simulink model "gyroPendulumBall"  (R2018a)
settings: Solver=FixedStepDiscrete  StartTime=0.0  StopTime=inf  FixedStep=timeStep  RelTol=1e-3
values from neighbouring files (symbols this model uses):
  K1 = [K1(1, :) K1(2, :)]    [alphaParallel.m]    (also in setup.m = lqr(Aw1, Bw1, diag([1, 1, 3, 1, 1, 1]), diag([6, 6])))
  K2 = lqr(Aw2, Bw2, diag([15, 1, 1, 5]), diag([15]))    [setup.m]
  K3 = lqr(Aw3, Bw3, diag([1, 1, 1, 1]), diag([1]))    [setup.m]
  modelParameters = rmfield(modelParameters, 'alph2')    [alphaParallel.m]    (also in setup.m)
  trajectory = [0.204039137261 -0.389047482528 0.184950739835 -0.34807965922 0.208093560422 -0.397377880713 0.182464301801 -0.343183800683 0.212362955443 -0.406162696705 0.180157605825 -0.338633761035 ... (832 elements, 4x208)]    [trajectory.mat]
  trajectoryTimeStep = 0.005    [setup.m]
  trajectoryToWalk = [0.20348839193 -0.387921068139 0.185314050902 -0.348794213842 0.206937106898 -0.395034683488 0.18313781068 -0.34450971149 0.210555704125 -0.402555806913 0.181086396317 -0.340463307968 ... (484 elements, 4x121)]    [trajectoryToWalk.mat]
  trajectoryWalk = [0.250192072849 -0.608547594051 0.394694165643 -0.613804432575 0.251033796696 -0.60716129389 0.397031433715 -0.614641196656 0.251771384595 -0.605603254171 0.399919372114 -0.616088285913 ... (1104 elements, 4x276)]    [trajectoryWalk.mat]
undefined symbols (not defined in the file or in its folder): DiscIntNeverNeededParam
libraries: simulink x4, dspindex x3, sharedtransform x1
settings Model: EnablePacing=on  PacingRate=2  Creator=Oleg  LastModifiedBy=sorok

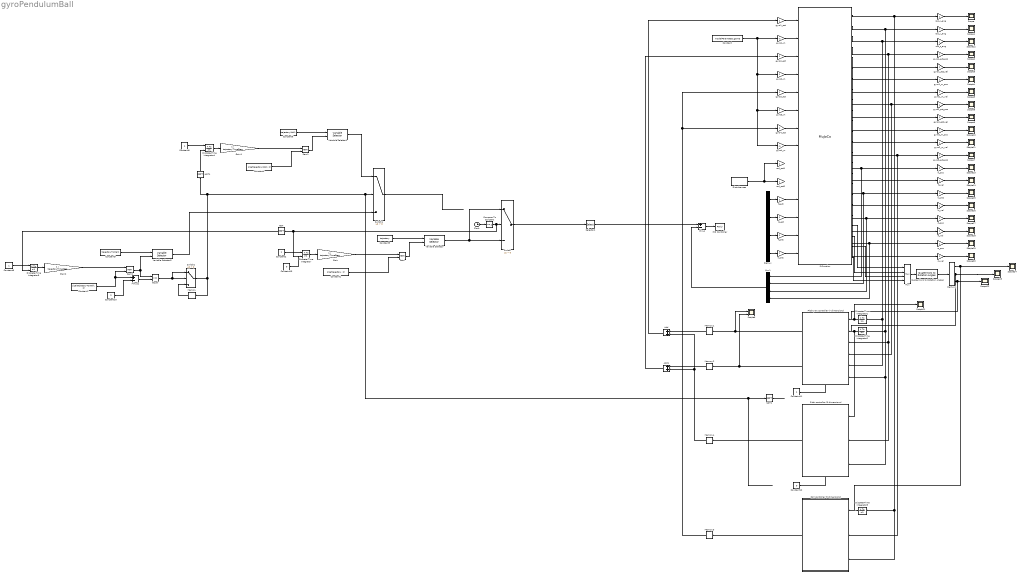
== system gyroPendulumBall ==
  Add : Sum
  Add1 : Sum
  Clock : Clock
  Compare To Constant : simulink/Logic and Bit Operations/Compare To Constant  relop=>=  const=2  OutDataTypeStr=boolean
  Constant : Constant  Value=modelParameters.gamD
  Constant1 : Constant  Value=size(trajectory, 2)
  Constant10 : Constant  Value=2
  Constant11 : Constant
  Constant12 : Constant  Value=0
  Constant13 : Constant  Value=0
  Constant2 : Constant  SampleTime=trajectoryTimeStep
  Constant3 : Constant  Value=trajectory
  Constant4 : Constant  Value=size(trajectoryWalk, 2)
  Constant5 : Constant  SampleTime=trajectoryTimeStep
  Constant6 : Constant  Value=trajectoryWalk
  Constant7 : Constant  Value=size(trajectoryToWalk, 2)
  Constant8 : Constant  SampleTime=trajectoryTimeStep
  Constant9 : Constant  Value=trajectoryToWalk
  Demux : Demux
  Demux1 : Demux  Outputs=3
  Discrete-Time Integrator : DiscreteIntegrator  ExternalReset=level  SampleTime=-1  ICPrevOutput=DiscIntNeverNeededParam  ICPrevScaledInput=DiscIntNeverNeededParam
  Discrete-Time Integrator1 : DiscreteIntegrator  SampleTime=-1  ICPrevOutput=DiscIntNeverNeededParam  ICPrevScaledInput=DiscIntNeverNeededParam
  Discrete-Time Integrator2 : DiscreteIntegrator  SampleTime=-1  ICPrevOutput=DiscIntNeverNeededParam  ICPrevScaledInput=DiscIntNeverNeededParam
  Discrete-Time Integrator3 : DiscreteIntegrator  SampleTime=-1  ICPrevOutput=DiscIntNeverNeededParam  ICPrevScaledInput=DiscIntNeverNeededParam
  Discrete-Time Integrator4 : DiscreteIntegrator  ExternalReset=level  SampleTime=-1  ICPrevOutput=DiscIntNeverNeededParam  ICPrevScaledInput=DiscIntNeverNeededParam
  Discrete-Time Integrator5 : DiscreteIntegrator  ExternalReset=level  SampleTime=-1  ICPrevOutput=DiscIntNeverNeededParam  ICPrevScaledInput=DiscIntNeverNeededParam
  Disturbances : Subsystem
  Equal : RelationalOperator  OutDataTypeStr=boolean  RndMeth=Simplest
  Gain : Gain  Gain=1 / trajectoryTimeStep
  Gain1 : Gain  Gain=1 / trajectoryTimeStep
  Gain2 : Gain  Gain=1 / trajectoryTimeStep
  Memory{,1..4} (5 alike) : Memory
  Minus : Sum  Inputs=+-
  Minus1 : Sum  Inputs=+-
  Mux : Mux
  Mux1 : Mux
  NOT : Logic  Operator=NOT  IconShape=distinctive  AllPortsSameDT=off  OutDataTypeStr=boolean
  NOT1 : Logic  Operator=NOT  IconShape=distinctive  AllPortsSameDT=off  OutDataTypeStr=boolean
  NOT2 : Logic  Operator=NOT  IconShape=distinctive  AllPortsSameDT=off  OutDataTypeStr=boolean
  PID Controller : simulink/Continuous/PID Controller  Controller=PD  TimeDomain=Discrete-time  SampleTime=-1  IntegratorMethod=Forward Euler  FilterMethod=Forward Euler  Form=Parallel  UseFilter=on  ControllerParametersSource=internal  P=300  I=1  D=300  N=100  InitialConditionSource=internal  InitialConditionForIntegrator=0  InitialConditionForFilter=0  ExternalReset=none  LimitOutput=off  UpperSaturationLimit=inf  LowerSaturationLimit=-inf  LinearizeAsGain=on  AntiWindupMode=none  Kb=1  TrackingMode=off  Kt=1  PParamMin=[]  PParamMax=[]  IParamMin=[]  IParamMax=[]  DParamMin=[]  DParamMax=[]  NParamMin=[]  NParamMax=[]  KbParamMin=[]  KbParamMax=[]  KtParamMin=[]  KtParamMax=[]  POutMin=[]  POutMax=[]  IOutMin=[]  IOutMax=[]  DOutMin=[]  DOutMax=[]  NOutMin=[]  NOutMax=[]  KbOutMin=[]  KbOutMax=[]  KtOutMin=[]  KtOutMax=[]  IntegratorOutMin=[]  IntegratorOutMax=[]  FilterOutMin=[]  FilterOutMax=[]  SumOutMin=[]  SumOutMax=[]  SumI1OutMin=[]  SumI1OutMax=[]  SumI2OutMin=[]  SumI2OutMax=[]  SumI3OutMin=[]  SumI3OutMax=[]  SumDOutMin=[]  SumDOutMax=[]  SaturationOutMin=[]  SaturationOutMax=[]  IntegratorContinuousStateAttributes=''  IntegratorStateMustResolveToSignalObject=off  IntegratorRTWStateStorageClass=Auto  FilterContinuousStateAttributes=''  FilterStateMustResolveToSignalObject=off  FilterRTWStateStorageClass=Auto  DifferentiatorICPrevScaledInput=0  DifferentiatorOutMin=[]  DifferentiatorOutMax=[]  FilterDiffOutCoefMin=[]  FilterDiffOutCoefMax=[]  SumDenOutMin=[]  SumDenOutMax=[]  SumNumOutMin=[]  SumNumOutMax=[]  ReciprocalOutMin=[]  ReciprocalOutMax=[]  DivideOutMin=[]  DivideOutMax=[]  TunerSelectOption=Transfer Function Based (PID Tuner App)
  Pitch controller (3 dimensions) : Subsystem
  Pitch-yaw controller (7 dimensions) : Subsystem
  Quaternions to Rotation Angles : sharedtransform/Quaternions to Rotation Angles  rotationOrder=XYZ  aMode=aMode
      settings: SourceProductBaseCode=AE
  Rem : Math  Operator=rem  SaturateOnIntegerOverflow=on
  Rem1 : Math  Operator=rem  SaturateOnIntegerOverflow=on
  Rem2 : Math  Operator=rem  SaturateOnIntegerOverflow=on
  Roll controller (3 dimensions) : Subsystem
  S-Function : S-Function  FunctionName=MuJoCo  SFunctionDeploymentMode=off  EnableBusSupport=off
  Scope{,1..5,7..24} (24 alike) : Scope
  Scope6 : Scope  NumInputPorts=2
  Selector1 : Selector  InputPortWidth=4  IndexOptions=Index vector (dialog)  Indices=[3 4 1 2]  OutputSizes=1
  Switch : Switch  Criteria=u2 > Threshold
  Switch1 : Switch  Criteria=u2 > Threshold
  Switch2 : Switch  Criteria=u2 > Threshold
  Variable Selector : dspindex/Variable Selector  NumInputs=1  rowsOrCols=Columns  IdxMode=Variable  Elements=[1 3]  ZerOneIdxMode=One-based  errmode=Clip Index  FillMode=on  FillValues=0
  Variable Selector1 : dspindex/Variable Selector  NumInputs=1  rowsOrCols=Columns  IdxMode=Variable  Elements=[1 3]  ZerOneIdxMode=One-based  errmode=Clip Index  FillMode=on  FillValues=0
  Variable Selector2 : dspindex/Variable Selector  NumInputs=1  rowsOrCols=Columns  IdxMode=Variable  Elements=[1 3]  ZerOneIdxMode=One-based  errmode=Clip Index  FillMode=on  FillValues=0
  gyro1_act : Gain
  gyro1_act_pos : Gain
  gyro1_act_vel : Gain
  gyro1_m : Gain  Gain=-1
  gyro1_m_pos : Gain
  gyro1_m_vel : Gain
  gyro2_act : Gain
  gyro2_act_pos : Gain
  gyro2_act_vel : Gain
  gyro2_m : Gain
  gyro2_m_pos : Gain
  gyro2_m_vel : Gain
  gyro3_act : Gain
  gyro3_act_pos : Gain
  gyro3_m : Gain
  gyro4_act : Gain
  gyro4_m : Gain  Gain=-1
  ls_act : Gain
  ls_pos : Gain
  ls_vel : Gain
  lt_act : Gain
  lt_pos : Gain
  lt_vel : Gain
  rod_act1 : Gain
  rod_act2 : Gain
  rod_x_ang : Gain
  rod_y_ang : Gain
  rod_z_ang : Gain
  rs_act : Gain
  rs_pos : Gain
  rs_vel : Gain
  rt_act : Gain
  rt_pos : Gain
  rt_vel : Gain
  wires:
  rod_x_ang/1 -> Scope/1
  gyro1_act_pos/1 -> Scope2/1
  rod_y_ang/1 -> Scope1/1
  gyro1_act_vel/1 -> Scope3/1
  gyro1_m_pos/1 -> Scope4/1
  gyro1_m_vel/1 -> Scope5/1
  Constant/1 -> gyro4_m/1, gyro3_m/1, gyro2_m/1, gyro1_m/1
  Pitch-yaw controller (7 dimensions)/1(alph1D) -> Scope6/1, Memory1/1
  Memory1/1 -> Add/1
  gyro1_m/1 -> S-Function/2
  gyro2_act/1 -> S-Function/3
  gyro2_m/1 -> S-Function/4
  gyro2_m_vel/1 -> Scope11/1
  gyro2_m_pos/1 -> Scope10/1
  gyro2_act_vel/1 -> Scope9/1
  gyro2_act_pos/1 -> Scope8/1
  rod_z_ang/1 -> Scope12/1
  Pitch-yaw controller (7 dimensions)/2(alph2D) -> Scope6/2, Memory2/1
  gyro1_act/1 -> S-Function/1
  Memory2/1 -> Add1/1
  Disturbances/1(Out) -> rod_act1/1, rod_act2/1
  Constant3/1 -> Variable Selector/1
  Variable Selector/1 -> Switch/1, Switch/3
  Discrete-Time Integrator/1 -> Gain/1
  Constant1/1 -> Rem/2
  Rem/1 -> Variable Selector/2
  Clock/1 -> Compare To Constant/1
  gyro3_m/1 -> S-Function/6
  gyro4_m/1 -> S-Function/8
  gyro3_act/1 -> S-Function/5
  gyro4_act/1 -> S-Function/7
  gyro3_act_pos/1 -> Scope7/1
  Memory3/1 -> gyro3_act/1, gyro4_act/1
  Compare To Constant/1 -> NOT/1, Switch/2
  Constant2/1 -> Discrete-Time Integrator/1
  Switch/1 -> Selector1/1
  S-Function/1 -> Discrete-Time Integrator3/1, Roll controller (3 dimensions)/3(sigmD), rod_x_ang/1
  S-Function/2 -> Discrete-Time Integrator2/1, Pitch controller (3 dimensions)/3(thetD), Pitch-yaw controller (7 dimensions)/6(thetD), rod_y_ang/1
  S-Function/3 -> Discrete-Time Integrator1/1, Pitch-yaw controller (7 dimensions)/5(psihD), rod_z_ang/1
  S-Function/4 -> Pitch-yaw controller (7 dimensions)/3(alph1), Pitch controller (3 dimensions)/2(alph1), gyro1_act_pos/1
  S-Function/5 -> gyro1_act_vel/1
  S-Function/6 -> gyro1_m_pos/1
  S-Function/7 -> gyro1_m_vel/1
  S-Function/8 -> Pitch-yaw controller (7 dimensions)/4(alph2), gyro2_act_pos/1
  S-Function/9 -> gyro2_act_vel/1
  S-Function/10 -> gyro2_m_pos/1
  S-Function/11 -> gyro2_m_vel/1
  S-Function/12 -> gyro3_act_pos/1, Roll controller (3 dimensions)/2(alph3)
  Gain/1 -> Rem/1
  Discrete-Time Integrator1/1 -> Scope21/1
  Discrete-Time Integrator2/1 -> Pitch controller (3 dimensions)/1(thet)
  Discrete-Time Integrator3/1 -> ?
  lt_act/1 -> S-Function/11
  ls_act/1 -> S-Function/12
  rt_act/1 -> S-Function/13
  rs_act/1 -> S-Function/14
  S-Function/14 -> lt_vel/1
  S-Function/13 -> Mux1/1, lt_pos/1
  S-Function/15 -> Mux1/2, ls_pos/1
  S-Function/16 -> ls_vel/1
  S-Function/17 -> Mux1/3, rt_pos/1
  S-Function/18 -> rt_vel/1
  S-Function/19 -> Mux1/4, rs_pos/1
  S-Function/20 -> rs_vel/1
  lt_pos/1 -> Scope13/1
  lt_vel/1 -> Scope14/1
  ls_pos/1 -> Scope15/1
  ls_vel/1 -> Scope16/1
  rt_pos/1 -> Scope17/1
  rt_vel/1 -> Scope18/1
  rs_pos/1 -> Scope19/1
  rs_vel/1 -> Scope20/1
  Demux/1 -> lt_act/1
  Demux/2 -> ls_act/1
  Demux/3 -> rt_act/1
  Demux/4 -> rs_act/1
  Minus/1 -> PID Controller/1
  Mux1/1 -> Minus/2
  Gain1/1 -> Rem1/1
  Constant5/1 -> Discrete-Time Integrator4/1
  Rem1/1 -> Variable Selector1/2
  Constant4/1 -> Rem1/2
  Discrete-Time Integrator4/1 -> Gain1/1
  Variable Selector1/1 -> Switch1/1
  Constant6/1 -> Variable Selector1/1
  NOT/1 -> Discrete-Time Integrator5/2
  Discrete-Time Integrator5/1 -> Gain2/1
  Constant8/1 -> Discrete-Time Integrator5/1
  Constant9/1 -> Variable Selector2/1
  Constant7/1 -> Minus1/1, Rem2/2
  Gain2/1 -> Rem2/1
  Rem2/1 -> Equal/1, Variable Selector2/2
  Equal/1 -> Switch2/1, Switch2/2
  Switch2/1 -> NOT1/1, Switch1/2, NOT2/1, Memory/1
  Memory/1 -> Switch2/3
  Switch1/1 -> ?
  Variable Selector2/1 -> Switch1/3
  NOT1/1 -> Discrete-Time Integrator4/2
  Minus1/1 -> Equal/2
  Constant10/1 -> Minus1/2
  NOT2/1 -> ?
  Pitch controller (3 dimensions)/1(alph1D) -> Memory4/1
  Memory4/1 -> Add/2, Add1/2
  Add/1 -> gyro1_act/1
  Add1/1 -> gyro2_act/1
  Constant11/1 -> Pitch-yaw controller (7 dimensions)/Enable
  Constant12/1 -> Pitch controller (3 dimensions)/Enable
  Selector1/1 -> Minus/1
  Constant13/1 -> Discrete-Time Integrator/2
  Roll controller (3 dimensions)/1(alph3D) -> Memory3/1
  Mux/1 -> Quaternions to Rotation Angles/1
  Quaternions to Rotation Angles/1 -> Demux1/1
  S-Function/21 -> Mux/1
  S-Function/22 -> Mux/2
  S-Function/23 -> Mux/3
  S-Function/24 -> Mux/4
  Demux1/3 -> Pitch-yaw controller (7 dimensions)/1(psih), Scope22/1
  Demux1/2 -> Scope23/1, Pitch-yaw controller (7 dimensions)/2(thet)
  Demux1/1 -> Scope24/1, Roll controller (3 dimensions)/1(sigm)

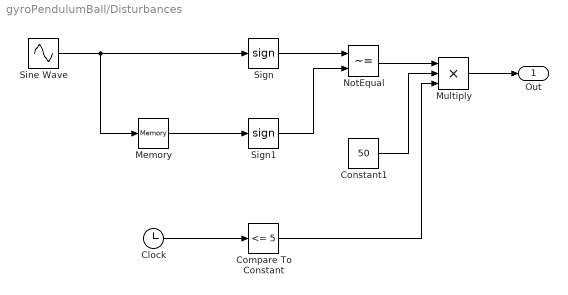
== system gyroPendulumBall/Disturbances ==
  Clock : Clock
  Compare To Constant : simulink/Logic and Bit Operations/Compare To Constant  relop=<=  const=5  OutDataTypeStr=boolean
  Constant1 : Constant  Value=50
  Memory : Memory
  Multiply : Product  Inputs=3
  NotEqual : RelationalOperator  Operator=~=  OutDataTypeStr=boolean  RndMeth=Simplest
  Sign : Signum
  Sign1 : Signum
  Sine Wave : Sin  Frequency=2  Phase=-0.5  SampleTime=0
  Out : Outport
  wires:
  Constant1/1 -> Multiply/2
  Multiply/1 -> Out/1
  Sign/1 -> NotEqual/1
  Sine Wave/1 -> Memory/1, Sign/1
  Clock/1 -> Compare To Constant/1
  NotEqual/1 -> Multiply/1
  Compare To Constant/1 -> Multiply/3
  Memory/1 -> Sign1/1
  Sign1/1 -> NotEqual/2

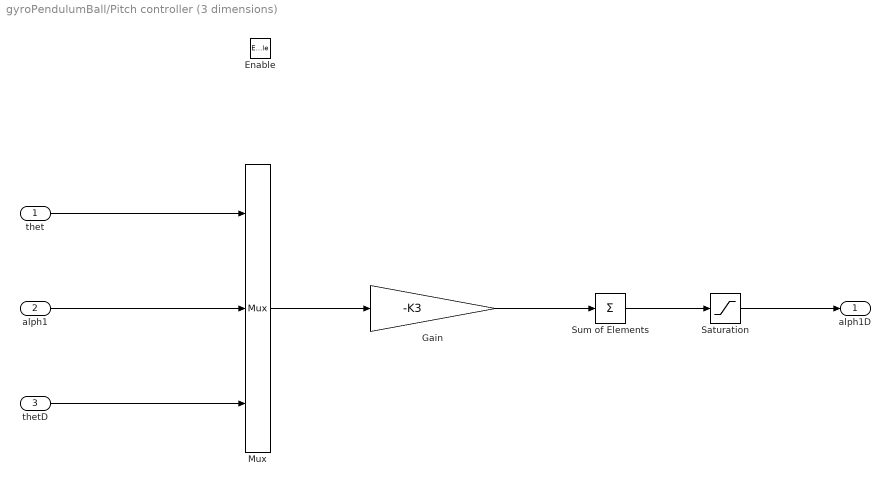
== system gyroPendulumBall/Pitch controller (3 dimensions) ==
  thet : Inport
  alph1 : Inport  Port=2
  thetD : Inport  Port=3
  Enable : EnablePort  StatesWhenEnabling=reset
  Gain : Gain  Gain=-K3
  Mux : Mux  Inputs=3
  Saturation : Saturate  UpperLimit=3  LowerLimit=-3
  Sum of Elements : Sum  Inputs=+
  alph1D : Outport
  wires:
  thetD/1 -> Mux/3
  thet/1 -> Mux/1
  alph1/1 -> Mux/2
  Mux/1 -> Gain/1
  Gain/1 -> Sum of Elements/1
  Sum of Elements/1 -> Saturation/1
  Saturation/1 -> alph1D/1

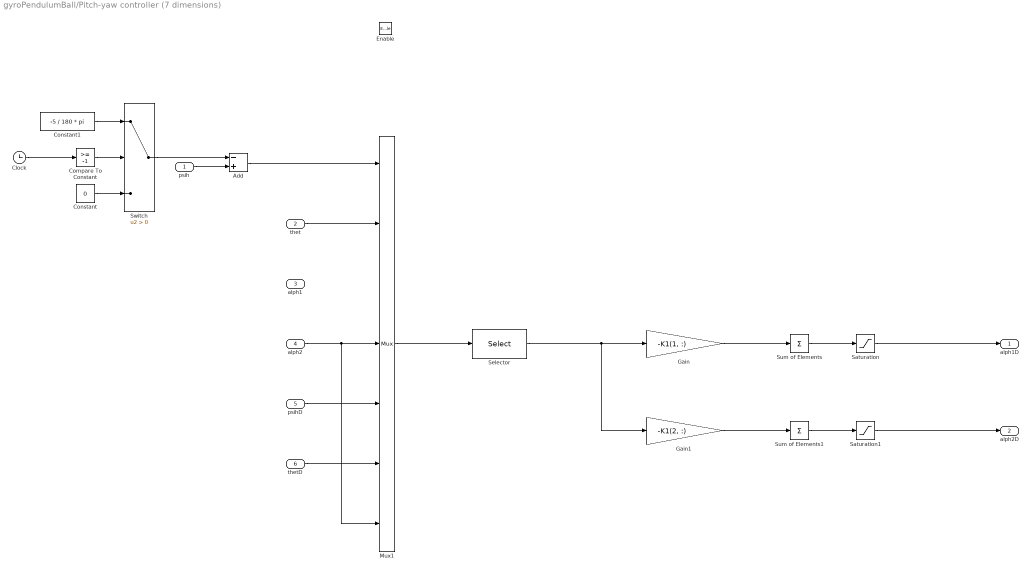
== system gyroPendulumBall/Pitch-yaw controller (7 dimensions) ==
  psih : Inport
  thet : Inport  Port=2
  alph1 : Inport  Port=3
  alph2 : Inport  Port=4
  psihD : Inport  Port=5
  thetD : Inport  Port=6
  Enable : EnablePort  StatesWhenEnabling=reset
  Add : Sum  Inputs=-+
  Clock : Clock
  Compare To Constant : simulink/Logic and Bit Operations/Compare To Constant  relop=>=  const=-1  OutDataTypeStr=boolean
  Constant : Constant  Value=0
  Constant1 : Constant  Value=-5 / 180 * pi
  Gain : Gain  Gain=-K1(1, :)
  Gain1 : Gain  Gain=-K1(2, :)
  Mux1 : Mux  Inputs=7
  Saturation : Saturate  UpperLimit=3  LowerLimit=-3
  Saturation1 : Saturate  UpperLimit=3  LowerLimit=-3
  Selector : Selector  NumberOfDimensions=2  InputPortWidth=7  IndexOptions=Index vector (dialog),Index vector (dialog)  Indices=1,[1 2 4 5 6 7]  OutputSizes=1,1
  Sum of Elements : Sum  Inputs=+
  Sum of Elements1 : Sum  Inputs=+
  Switch : Switch  Criteria=u2 > Threshold
  alph1D : Outport
  alph2D : Outport  Port=2
  wires:
  Gain/1 -> Sum of Elements/1
  Sum of Elements/1 -> Saturation/1
  Saturation/1 -> alph1D/1
  Gain1/1 -> Sum of Elements1/1
  Sum of Elements1/1 -> Saturation1/1
  Saturation1/1 -> alph2D/1
  Clock/1 -> Compare To Constant/1
  Compare To Constant/1 -> Switch/2
  Add/1 -> Mux1/1
  Constant/1 -> Switch/3
  Constant1/1 -> Switch/1
  psih/1 -> Add/2
  thet/1 -> Mux1/2
  psihD/1 -> Mux1/5
  thetD/1 -> Mux1/6
  Mux1/1 -> Selector/1
  alph2/1 -> Mux1/7, Mux1/4
  Selector/1 -> Gain/1, Gain1/1
  Switch/1 -> Add/1

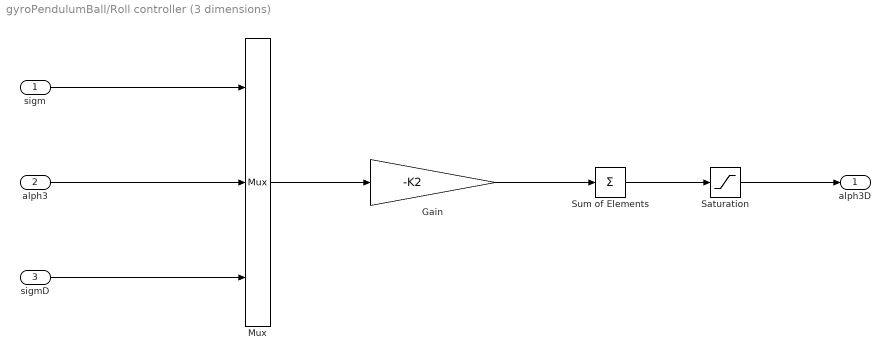
== system gyroPendulumBall/Roll controller (3 dimensions) ==
  sigm : Inport
  alph3 : Inport  Port=2
  sigmD : Inport  Port=3
  Gain : Gain  Gain=-K2
  Mux : Mux  Inputs=3
  Saturation : Saturate  UpperLimit=3  LowerLimit=-3
  Sum of Elements : Sum  Inputs=+
  alph3D : Outport
  wires:
  Saturation/1 -> alph3D/1
  Sum of Elements/1 -> Saturation/1
  Gain/1 -> Sum of Elements/1
  Mux/1 -> Gain/1
  alph3/1 -> Mux/2
  sigm/1 -> Mux/1
  sigmD/1 -> Mux/3
